simulink model "PID_Sim_2012a"  (R2012a)
settings: Solver=ode8  SolverMode=SingleTasking  StartTime=0.0  StopTime=30  FixedStep=1e-3  RelTol=1e-3
undefined symbols (not defined in the file): d_initial, x_initial, x_soll
libraries: simulink x1
settings Model: CovMetricSettings=dwe  CovHtmlReporting=off  covSaveCumulativeToWorkspaceVar=off  CovSaveSingleToWorkspaceVar=off  CovExternalEMLEnable=on  Creator=Naresh  LastModifiedBy=Naresh
settings DataIOCC: SaveFormat=StructureWithTime  ReturnWorkspaceOutputs=off
settings OptimizationCC: LifeSpan=inf  SimCompilerOptimization=Off
settings DebuggingCC: FcnCallInpInsideContextMsg=Enable All
settings HardwareCC: ProdWordSize=32  ProdHWDeviceType=Specified
settings RTWCC: RTWCompilerOptimization=Off
settings GRTTargetCC: CodeReplacementLibrary=C99 (ISO)  CPPClassGenCompliant=off

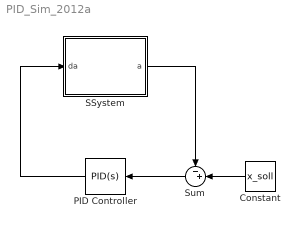
== system PID_Sim_2012a ==
  Constant : Constant  Value=x_soll
  PID Controller : simulink/Continuous/PID Controller  Controller=PID  Form=Parallel  TimeDomain=Continuous-time  SampleTime=-1  IntegratorMethod=Forward Euler  FilterMethod=Forward Euler  ControllerParametersSource=internal  P=141.186500513683  I=10.2563359586177  D=88.1677030624935  UseFilter=on  N=996.227139608466  InitialConditionSource=internal  InitialConditionForIntegrator=0  InitialConditionForFilter=0  DifferentiatorICPrevScaledInput=0  ExternalReset=none  TrackingMode=off  Kt=1  LimitOutput=on  UpperSaturationLimit=80  LowerSaturationLimit=-80  LinearizeAsGain=off  AntiWindupMode=none  Kb=1  POutMin=[]  POutMax=[]  IOutMin=[]  IOutMax=[]  DOutMin=[]  DOutMax=[]  NOutMin=[]  NOutMax=[]  SumOutMin=[]  SumOutMax=[]  SaturationOutMin=[]  SaturationOutMax=[]  PParamMin=[]  PParamMax=[]  IParamMin=[]  IParamMax=[]  DParamMin=[]  DParamMax=[]  NParamMin=[]  NParamMax=[]  KbParamMin=[]  KbParamMax=[]  KtParamMin=[]  KtParamMax=[]  KbOutMin=[]  KbOutMax=[]  KtOutMin=[]  KtOutMax=[]  IntegratorOutMin=[]  IntegratorOutMax=[]  FilterOutMin=[]  FilterOutMax=[]  SumI1OutMin=[]  SumI1OutMax=[]  SumI2OutMin=[]  SumI2OutMax=[]  SumI3OutMin=[]  SumI3OutMax=[]  SumDOutMin=[]  SumDOutMax=[]  DifferentiatorOutMin=[]  DifferentiatorOutMax=[]  IntegratorContinuousStateAttributes=''  IntegratorStateMustResolveToSignalObject=off  IntegratorRTWStateStorageClass=Auto  FilterContinuousStateAttributes=''  FilterStateMustResolveToSignalObject=off  FilterRTWStateStorageClass=Auto
  SSystem : Subsystem
  Sum : Sum  Inputs=-+|
  wires:
  SSystem/1(a) -> Sum/1
  Sum/1 -> PID Controller/1
  PID Controller/1 -> SSystem/1(da)
  Constant/1 -> Sum/2

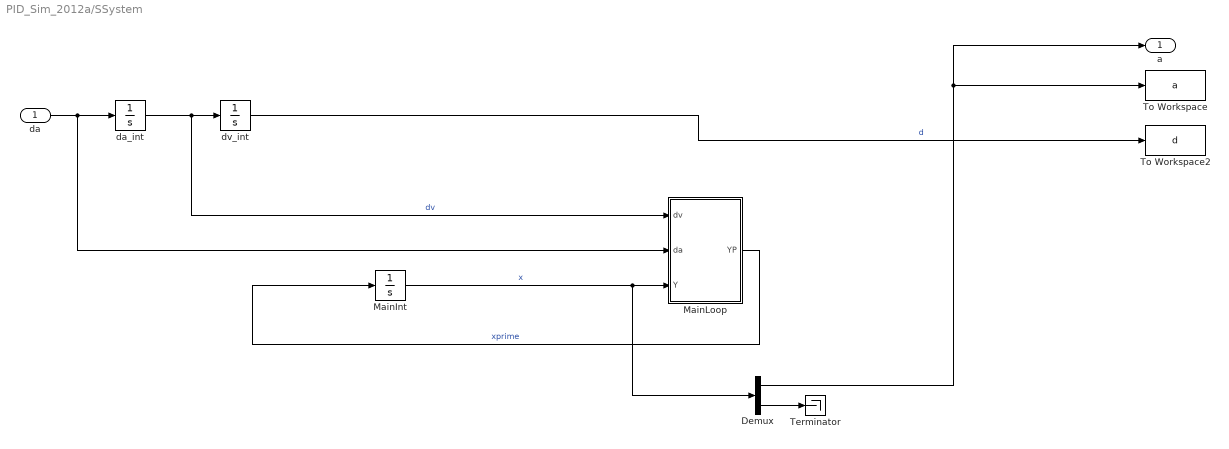
== system PID_Sim_2012a/SSystem ==
  da : Inport
  Demux : Demux  Outputs=2
  MainInt : Integrator  InitialCondition=x_initial
  MainLoop : MATLAB Function  TreatAsAtomicUnit=on
      settings: PermitHierarchicalResolution=ParametersOnly
  Terminator : Terminator
  To Workspace : ToWorkspace  VariableName=a  SaveFormat=Timeseries  SampleTime=-1
  To Workspace2 : ToWorkspace  VariableName=d  SaveFormat=Timeseries  SampleTime=-1
  da_int : Integrator  InitialCondition=d_initial(2)
  dv_int : Integrator  InitialCondition=d_initial(1)
  a : Outport
  wires:
  da/1 -> MainLoop/2(da), da_int/1
  MainInt/1 -> Demux/1, MainLoop/3(Y)  "x"
  da_int/1 -> MainLoop/1(dv), dv_int/1  "dv"
  MainLoop/1(YP) -> MainInt/1  "xprime"
  dv_int/1 -> To Workspace2/1  "d"
  Demux/2 -> Terminator/1
  Demux/1 -> a/1, To Workspace/1

== matlab function PID_Sim_2012a/SSystem/MainLoop ==
  data: dv input; YP output; da input; Y input
function YP = MainLoop(dv,da,Y)
    g = 9.81;
    L = 10;
    m=2;
    lambda=1;

    YP = zeros(2,1);

    YP(1) = Y(2);
    YP(2) = (-L * lambda * Y(2) - dv * cos(Y(1)) * lambda - da * cos(Y(1)) * m - sin(Y(1)) * g * m) / L / m;

end
